simulink library "halout"  (R2021b)
settings: Solver=VariableStepAuto  StartTime=0.0  StopTime=10.0  RelTol=1e-3
undefined symbols (not defined in the file): C_TASK_5MS_S, FALSE, KHAL_CAN1FDAPS3E2E_flg, KHAL_CAN1FDAPS3TxReq_flg, KHAL_CAN1FDVCU2E2E_flg, KHAL_CAN1FDVCU2TxReq_flg, KHAL_CAN1FDVCU3E2E_flg, KHAL_CAN1FDVCU3TxReq_flg, KHAL_CAN1TxReq_flg, KHAL_CAN2TxReq_flg, KHAL_CAN3FDVCU1TxReq_flg, KHAL_CAN3FDVCU2E2E_flg, KHAL_CAN3FDVCU2TxReq_flg, KHAL_CAN3TxReq_flg, KHAL_CAN4FDVCU1E2E_flg, KHAL_CAN4FDVCU1TxReq_flg, KHAL_CAN4TxReq_flg, KHAL_CAN5TxReq_flg, ONE_INT, TRUE, ZERO_INT
libraries: FVT_lib x383, simulink x179
(part 10 of 20)

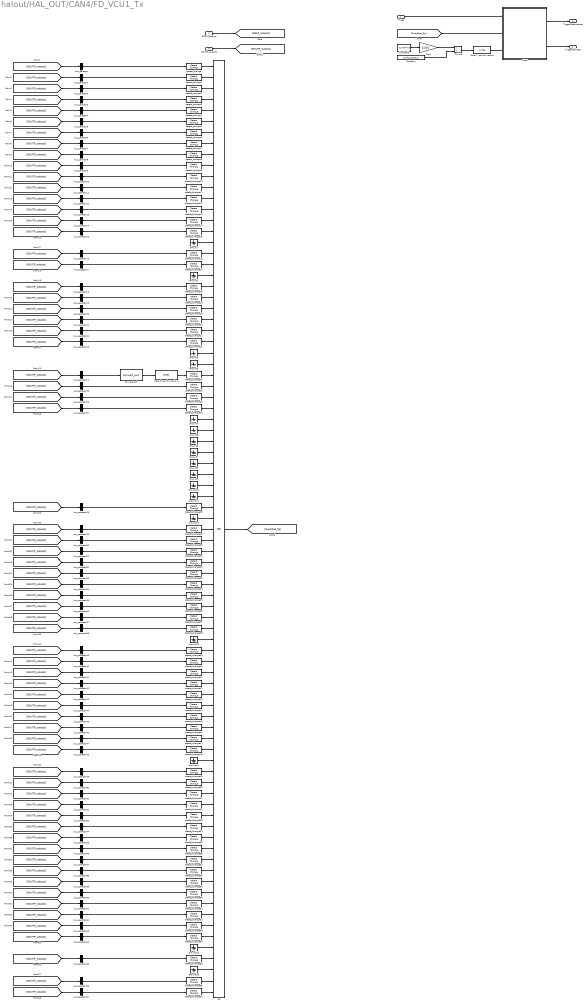
== system halout/HAL_OUT/CAN4/FD_VCU1_Tx ==
  TxReq : Inport
  BSCP_outputs : Inport  Port=2  OutDataTypeStr=Bus: BSCP_outputs
  BOUTP_outputs : Inport  Port=3  OutDataTypeStr=Bus: BOUTP_outputs
  Chart : Stateflow chart  TreatAsAtomicUnit=on
  Constant : Constant  Value=C_TASK_5MS_S
  Constant3 : Constant  Value=CycleTime
  Data Type Conversion : DataTypeConversion  OutDataTypeStr=uint16
  Data Type Conversion1 : DataTypeConversion  OutDataTypeStr=uint8
  Divide : Product  Inputs=*/
  Gain : Gain  Gain=0.001
  Ground{,1..16} (17 alike) : Ground
  OR : Logic  Operator=OR  Inputs=85  AllPortsSameDT=off  OutDataTypeStr=boolean
  bus_selector : BusSelector  OutputSignals=VOUTP_AllDoorSW_flg
  bus_selector1 : BusSelector  OutputSignals=VOUTP_AmbLightBreath1_flg
  bus_selector10 : BusSelector  OutputSignals=VOUTP_AntitheftSeatFlod_flg
  bus_selector11 : BusSelector  OutputSignals=VOUTP_AntitheftSta_enum
  bus_selector12 : BusSelector  OutputSignals=VOUTP_BCMBuzzerReq_flg
  bus_selector13 : BusSelector  OutputSignals=VOUTP_BCMDoorLockSta_flg
  bus_selector14 : BusSelector  OutputSignals=VOUTP_BrakeLamp_flg
  bus_selector15 : BusSelector  OutputSignals=VOUTP_CCCtrlSta_enum
  bus_selector16 : BusSelector  OutputSignals=VOUTP_CTDCtrl_enum
  bus_selector17 : BusSelector  OutputSignals=VOUTP_CTDLockSW_flg
  bus_selector18 : BusSelector  OutputSignals=VOUTP_CrashDetd_flg
  bus_selector19 : BusSelector  OutputSignals=VOUTP_CtrlDrPwrStbA2_flg
  bus_selector2 : BusSelector  OutputSignals=VOUTP_AmbLightBreath2_flg
  bus_selector20 : BusSelector  OutputSignals=VOUTP_CtrlFrBMSCCUCIR_flg
  bus_selector21 : BusSelector  OutputSignals=VOUTP_CtrlFrEDUINVERTER_flg
  bus_selector22 : BusSelector  OutputSignals=VOUTP_CtrlFrRC1_flg
  bus_selector23 : BusSelector  OutputSignals=VOUTP_CtrlFrPwrStbA1P_flg
  bus_selector24 : BusSelector  OutputSignals=VOUTP_Dimmer_pct
  bus_selector25 : BusSelector  OutputSignals=VOUTP_DimmerEN_flg
  bus_selector26 : BusSelector  OutputSignals=VOUTP_DoorLockIND_flg
  bus_selector27 : BusSelector  OutputSignals=VOUTP_DrDoorSW_flg
  bus_selector28 : BusSelector  OutputSignals=VOUTP_FrChargingDoorCtrl_enum
  bus_selector29 : BusSelector  OutputSignals=VOUTP_FrWiperH_flg
  bus_selector3 : BusSelector  OutputSignals=VOUTP_AmbLightBreath3_flg
  bus_selector30 : BusSelector  OutputSignals=VOUTP_FrWiperL_flg
  bus_selector31 : BusSelector  OutputSignals=VOUTP_HWResetSta_enum
  bus_selector32 : BusSelector  OutputSignals=VOUTP_HBeam_flg
  bus_selector33 : BusSelector  OutputSignals=VOUTP_HazardSW_flg
  bus_selector34 : BusSelector  OutputSignals=VOUTP_HoodSW_flg
  bus_selector35 : BusSelector  OutputSignals=VOUTP_HornCtrl_flg
  bus_selector36 : BusSelector  OutputSignals=VOUTP_LBSD_flg
  bus_selector37 : BusSelector  OutputSignals=VOUTP_LDRL_flg
  bus_selector38 : BusSelector  OutputSignals=VOUTP_LTurnLP_flg
  bus_selector39 : BusSelector  OutputSignals=VOUTP_LBeam_flg
  bus_selector4 : BusSelector  OutputSignals=VOUTP_AmbLightBrightness1_enum
  bus_selector40 : BusSelector  OutputSignals=VOUTP_LampPwr_flg
  bus_selector41 : BusSelector  OutputSignals=VOUTP_LockSetting_flg
  bus_selector42 : BusSelector  OutputSignals=VOUTP_MSACtrlSta_enum
  bus_selector43 : BusSelector  OutputSignals=VOUTP_MirrorCtrl_enum
  bus_selector44 : BusSelector  OutputSignals=VOUTP_MirrorDefog_flg
  bus_selector45 : BusSelector  OutputSignals=VOUTP_PosLamp_flg
  bus_selector46 : BusSelector  OutputSignals=VOUTP_PsDoorSW_flg
  bus_selector47 : BusSelector  OutputSignals=VOUTP_PowerSta_enum
  bus_selector48 : BusSelector  OutputSignals=VOUTP_RBSD_flg
  bus_selector49 : BusSelector  OutputSignals=VOUTP_RDRL_flg
  bus_selector5 : BusSelector  OutputSignals=VOUTP_AmbLightBrightness2_enum
  bus_selector50 : BusSelector  OutputSignals=VOUTP_RLDoorSW_flg
  bus_selector51 : BusSelector  OutputSignals=VOUTP_RRDoorSW_flg
  bus_selector52 : BusSelector  OutputSignals=VOUTP_RTurnLP_flg
  bus_selector53 : BusSelector  OutputSignals=VOUTP_ReBrakeLPReq_flg
  bus_selector54 : BusSelector  OutputSignals=VOUTP_ReverseLamp_flg
  bus_selector55 : BusSelector  OutputSignals=VOUTP_RoomLampH_flg
  bus_selector56 : BusSelector  OutputSignals=VOUTP_RoomLampL_flg
  bus_selector57 : BusSelector  OutputSignals=VOUTP_RrChargingDoorCtrl_enum
  bus_selector58 : BusSelector  OutputSignals=VOUTP_RrDefog_flg
  bus_selector59 : BusSelector  OutputSignals=VOUTP_RrFogLamp_flg
  bus_selector6 : BusSelector  OutputSignals=VOUTP_AmbLightBrightness3_enum
  bus_selector60 : BusSelector  OutputSignals=VOUTP_RrWiper_flg
  bus_selector61 : BusSelector  OutputSignals=VOUTP_ShiftGearPosn_enum
  bus_selector62 : BusSelector  OutputSignals=VOUTP_TailgateHDSW_flg
  bus_selector63 : BusSelector  OutputSignals=VOUTP_TailgateRemote_enum
  bus_selector64 : BusSelector  OutputSignals=VOUTP_TailgateSW_flg
  bus_selector65 : BusSelector  OutputSignals=VOUTP_TrunkRel_flg
  bus_selector66 : BusSelector  OutputSignals=VOUTP_WasherCtrl_enum
  bus_selector67 : BusSelector  OutputSignals=VOUTP_WiperFixMode_flg
  bus_selector7 : BusSelector  OutputSignals=VOUTP_AmbLightColor1_enum
  bus_selector8 : BusSelector  OutputSignals=VOUTP_AmbLightColor2_enum
  bus_selector9 : BusSelector  OutputSignals=VOUTP_AmbLightColor3_enum
  convert_out : FVT_lib/hal/convert_out  gain=1  offset=0
  detect_change{,1..67} (68 alike) : simulink/Logic and Bit Operations/Detect Change  vinit=0  OutDataTypeStr=boolean
  TriggerDataUpdate : Outport
  TriggerCallCDD : Outport  Port=2
  wires:
  Data Type Conversion/1 -> Chart/3(CycleCnt)
  TxReq/1 -> Chart/1(TxReq)
  [EventReq_flg] -> Chart/2(EventReq)
  Constant/1 -> Divide/2
  Divide/1 -> Data Type Conversion/1
  Gain/1 -> Divide/1
  Constant3/1 -> Gain/1
  BSCP_outputs/1 -> [BSCP_outputs]
  BOUTP_outputs/1 -> [BOUTP_outputs]
  OR/1 -> [EventReq_flg]
  detect_change/1 -> OR/1
  bus_selector/1 -> detect_change/1  "<VOUTP_AllDoorSW_flg>"
  [BOUTP_outputs] -> bus_selector/1
  detect_change1/1 -> OR/2
  bus_selector1/1 -> detect_change1/1  "<VOUTP_AmbLightBreath1_flg>"
  [BOUTP_outputs] -> bus_selector1/1
  detect_change2/1 -> OR/3
  bus_selector2/1 -> detect_change2/1  "<VOUTP_AmbLightBreath2_flg>"
  [BOUTP_outputs] -> bus_selector2/1
  detect_change3/1 -> OR/4
  bus_selector3/1 -> detect_change3/1  "<VOUTP_AmbLightBreath3_flg>"
  [BOUTP_outputs] -> bus_selector3/1
  detect_change4/1 -> OR/5
  bus_selector4/1 -> detect_change4/1  "<VOUTP_AmbLightBrightness1_enum>"
  [BOUTP_outputs] -> bus_selector4/1
  detect_change5/1 -> OR/6
  bus_selector5/1 -> detect_change5/1  "<VOUTP_AmbLightBrightness2_enum>"
  [BOUTP_outputs] -> bus_selector5/1
  detect_change6/1 -> OR/7
  bus_selector6/1 -> detect_change6/1  "<VOUTP_AmbLightBrightness3_enum>"
  [BOUTP_outputs] -> bus_selector6/1
  detect_change7/1 -> OR/8
  bus_selector7/1 -> detect_change7/1  "<VOUTP_AmbLightColor1_enum>"
  [BOUTP_outputs] -> bus_selector7/1
  detect_change8/1 -> OR/9
  bus_selector8/1 -> detect_change8/1  "<VOUTP_AmbLightColor2_enum>"
  [BOUTP_outputs] -> bus_selector8/1
  detect_change9/1 -> OR/10
  bus_selector9/1 -> detect_change9/1  "<VOUTP_AmbLightColor3_enum>"
  [BOUTP_outputs] -> bus_selector9/1
  detect_change10/1 -> OR/11
  bus_selector10/1 -> detect_change10/1  "<VOUTP_AntitheftSeatFlod_flg>"
  [BOUTP_outputs] -> bus_selector10/1
  detect_change11/1 -> OR/12
  bus_selector11/1 -> detect_change11/1  "<VOUTP_AntitheftSta_enum>"
  [BOUTP_outputs] -> bus_selector11/1
  detect_change12/1 -> OR/13
  bus_selector12/1 -> detect_change12/1  "<VOUTP_BCMBuzzerReq_flg>"
  [BOUTP_outputs] -> bus_selector12/1
  detect_change13/1 -> OR/14
  bus_selector13/1 -> detect_change13/1  "<VOUTP_BCMDoorLockSta_flg>"
  [BOUTP_outputs] -> bus_selector13/1
  detect_change14/1 -> OR/15
  bus_selector14/1 -> detect_change14/1  "<VOUTP_BrakeLamp_flg>"
  [BOUTP_outputs] -> bus_selector14/1
  detect_change15/1 -> OR/16
  bus_selector15/1 -> detect_change15/1  "<VOUTP_CCCtrlSta_enum>"
  [BOUTP_outputs] -> bus_selector15/1
  Ground/1 -> OR/17
  detect_change16/1 -> OR/18
  bus_selector16/1 -> detect_change16/1  "<VOUTP_CTDCtrl_enum>"
  [BOUTP_outputs] -> bus_selector16/1
  detect_change17/1 -> OR/19
  bus_selector17/1 -> detect_change17/1  "<VOUTP_CTDLockSW_flg>"
  [BOUTP_outputs] -> bus_selector17/1
  Ground1/1 -> OR/20
  detect_change18/1 -> OR/21
  bus_selector18/1 -> detect_change18/1  "<VOUTP_CrashDetd_flg>"
  [BOUTP_outputs] -> bus_selector18/1
  detect_change19/1 -> OR/22
  bus_selector19/1 -> detect_change19/1  "<VOUTP_CtrlDrPwrStbA2_flg>"
  [BOUTP_outputs] -> bus_selector19/1
  detect_change20/1 -> OR/23
  bus_selector20/1 -> detect_change20/1  "<VOUTP_CtrlFrBMSCCUCIR_flg>"
  [BOUTP_outputs] -> bus_selector20/1
  detect_change21/1 -> OR/24
  bus_selector21/1 -> detect_change21/1  "<VOUTP_CtrlFrEDUINVERTER_flg>"
  [BOUTP_outputs] -> bus_selector21/1
  detect_change22/1 -> OR/25
  bus_selector22/1 -> detect_change22/1  "<VOUTP_CtrlFrRC1_flg>"
  [BOUTP_outputs] -> bus_selector22/1
  detect_change23/1 -> OR/26
  bus_selector23/1 -> detect_change23/1  "<VOUTP_CtrlFrPwrStbA1P_flg>"
  [BOUTP_outputs] -> bus_selector23/1
  Ground2/1 -> OR/27
  Ground3/1 -> OR/28
  detect_change24/1 -> OR/29
  Data Type Conversion1/1 -> detect_change24/1
  convert_out/1 -> Data Type Conversion1/1
  bus_selector24/1 -> convert_out/1  "<VOUTP_Dimmer_pct>"
  [BOUTP_outputs] -> bus_selector24/1
  detect_change25/1 -> OR/30
  bus_selector25/1 -> detect_change25/1  "<VOUTP_DimmerEN_flg>"
  [BOUTP_outputs] -> bus_selector25/1
  detect_change26/1 -> OR/31
  bus_selector26/1 -> detect_change26/1  "<VOUTP_DoorLockIND_flg>"
  [BOUTP_outputs] -> bus_selector26/1
  detect_change27/1 -> OR/32
  bus_selector27/1 -> detect_change27/1  "<VOUTP_DrDoorSW_flg>"
  [BOUTP_outputs] -> bus_selector27/1
  Ground4/1 -> OR/33
  Ground5/1 -> OR/34
  Ground6/1 -> OR/35
  Ground7/1 -> OR/36
  Ground8/1 -> OR/37
  Ground9/1 -> OR/38
  Ground10/1 -> OR/39
  Ground11/1 -> OR/40
  detect_change28/1 -> OR/41
  bus_selector28/1 -> detect_change28/1  "<VOUTP_FrChargingDoorCtrl_enum>"
  [BOUTP_outputs] -> bus_selector28/1
  Ground12/1 -> OR/42
  detect_change29/1 -> OR/43
  bus_selector29/1 -> detect_change29/1  "<VOUTP_FrWiperH_flg>"
  [BOUTP_outputs] -> bus_selector29/1
  detect_change30/1 -> OR/44
  bus_selector30/1 -> detect_change30/1  "<VOUTP_FrWiperL_flg>"
  [BOUTP_outputs] -> bus_selector30/1
  detect_change31/1 -> OR/45
  bus_selector31/1 -> detect_change31/1  "<VOUTP_HWResetSta_enum>"
  [BOUTP_outputs] -> bus_selector31/1
  detect_change32/1 -> OR/46
  bus_selector32/1 -> detect_change32/1  "<VOUTP_HBeam_flg>"
  [BOUTP_outputs] -> bus_selector32/1
  detect_change33/1 -> OR/47
  bus_selector33/1 -> detect_change33/1  "<VOUTP_HazardSW_flg>"
  [BOUTP_outputs] -> bus_selector33/1
  detect_change34/1 -> OR/48
  bus_selector34/1 -> detect_change34/1  "<VOUTP_HoodSW_flg>"
  [BOUTP_outputs] -> bus_selector34/1
  detect_change35/1 -> OR/49
  bus_selector35/1 -> detect_change35/1  "<VOUTP_HornCtrl_flg>"
  [BOUTP_outputs] -> bus_selector35/1
  detect_change36/1 -> OR/50
  bus_selector36/1 -> detect_change36/1  "<VOUTP_LBSD_flg>"
  [BOUTP_outputs] -> bus_selector36/1
  detect_change37/1 -> OR/51
  bus_selector37/1 -> detect_change37/1  "<VOUTP_LDRL_flg>"
  [BOUTP_outputs] -> bus_selector37/1
  detect_change38/1 -> OR/52
  bus_selector38/1 -> detect_change38/1  "<VOUTP_LTurnLP_flg>"
  [BOUTP_outputs] -> bus_selector38/1
  Ground13/1 -> OR/53
  detect_change39/1 -> OR/54
  bus_selector39/1 -> detect_change39/1  "<VOUTP_LBeam_flg>"
  [BOUTP_outputs] -> bus_selector39/1
  detect_change40/1 -> OR/55
  bus_selector40/1 -> detect_change40/1  "<VOUTP_LampPwr_flg>"
  [BOUTP_outputs] -> bus_selector40/1
  detect_change41/1 -> OR/56
  bus_selector41/1 -> detect_change41/1  "<VOUTP_LockSetting_flg>"
  [BOUTP_outputs] -> bus_selector41/1
  detect_change42/1 -> OR/57
  bus_selector42/1 -> detect_change42/1  "<VOUTP_MSACtrlSta_enum>"
  [BOUTP_outputs] -> bus_selector42/1
  detect_change43/1 -> OR/58
  bus_selector43/1 -> detect_change43/1  "<VOUTP_MirrorCtrl_enum>"
  [BOUTP_outputs] -> bus_selector43/1
  detect_change44/1 -> OR/59
  bus_selector44/1 -> detect_change44/1  "<VOUTP_MirrorDefog_flg>"
  [BOUTP_outputs] -> bus_selector44/1
  detect_change45/1 -> OR/60
  bus_selector45/1 -> detect_change45/1  "<VOUTP_PosLamp_flg>"
  [BOUTP_outputs] -> bus_selector45/1
  detect_change46/1 -> OR/61
  bus_selector46/1 -> detect_change46/1  "<VOUTP_PsDoorSW_flg>"
  [BOUTP_outputs] -> bus_selector46/1
  detect_change47/1 -> OR/62
  bus_selector47/1 -> detect_change47/1  "<VOUTP_PowerSta_enum>"
  [BOUTP_outputs] -> bus_selector47/1
  detect_change48/1 -> OR/63
  bus_selector48/1 -> detect_change48/1  "<VOUTP_RBSD_flg>"
  [BOUTP_outputs] -> bus_selector48/1
  Ground14/1 -> OR/64
  detect_change49/1 -> OR/65
  bus_selector49/1 -> detect_change49/1  "<VOUTP_RDRL_flg>"
  [BOUTP_outputs] -> bus_selector49/1
  detect_change50/1 -> OR/66
  bus_selector50/1 -> detect_change50/1  "<VOUTP_RLDoorSW_flg>"
  [BOUTP_outputs] -> bus_selector50/1
  detect_change51/1 -> OR/67
  bus_selector51/1 -> detect_change51/1  "<VOUTP_RRDoorSW_flg>"
  [BOUTP_outputs] -> bus_selector51/1
  detect_change52/1 -> OR/68
  bus_selector52/1 -> detect_change52/1  "<VOUTP_RTurnLP_flg>"
  [BOUTP_outputs] -> bus_selector52/1
  detect_change53/1 -> OR/69
  bus_selector53/1 -> detect_change53/1  "<VOUTP_ReBrakeLPReq_flg>"
  [BOUTP_outputs] -> bus_selector53/1
  detect_change54/1 -> OR/70
  bus_selector54/1 -> detect_change54/1  "<VOUTP_ReverseLamp_flg>"
  [BOUTP_outputs] -> bus_selector54/1
  detect_change55/1 -> OR/71
  bus_selector55/1 -> detect_change55/1  "<VOUTP_RoomLampH_flg>"
  [BOUTP_outputs] -> bus_selector55/1
  detect_change56/1 -> OR/72
  bus_selector56/1 -> detect_change56/1  "<VOUTP_RoomLampL_flg>"
  [BOUTP_outputs] -> bus_selector56/1
  detect_change57/1 -> OR/73
  bus_selector57/1 -> detect_change57/1  "<VOUTP_RrChargingDoorCtrl_enum>"
  [BOUTP_outputs] -> bus_selector57/1
  detect_change58/1 -> OR/74
  bus_selector58/1 -> detect_change58/1  "<VOUTP_RrDefog_flg>"
  [BOUTP_outputs] -> bus_selector58/1
  detect_change59/1 -> OR/75
  bus_selector59/1 -> detect_change59/1  "<VOUTP_RrFogLamp_flg>"
  [BOUTP_outputs] -> bus_selector59/1
  detect_change60/1 -> OR/76
  bus_selector60/1 -> detect_change60/1  "<VOUTP_RrWiper_flg>"
  [BOUTP_outputs] -> bus_selector60/1
  detect_change61/1 -> OR/77
  bus_selector61/1 -> detect_change61/1  "<VOUTP_ShiftGearPosn_enum>"
  [BOUTP_outputs] -> bus_selector61/1
  detect_change62/1 -> OR/78
  bus_selector62/1 -> detect_change62/1  "<VOUTP_TailgateHDSW_flg>"
  [BOUTP_outputs] -> bus_selector62/1
  detect_change63/1 -> OR/79
  bus_selector63/1 -> detect_change63/1  "<VOUTP_TailgateRemote_enum>"
  [BOUTP_outputs] -> bus_selector63/1
  detect_change64/1 -> OR/80
  bus_selector64/1 -> detect_change64/1  "<VOUTP_TailgateSW_flg>"
  [BOUTP_outputs] -> bus_selector64/1
  Ground15/1 -> OR/81
  detect_change65/1 -> OR/82
  bus_selector65/1 -> detect_change65/1  "<VOUTP_TrunkRel_flg>"
  [BOUTP_outputs] -> bus_selector65/1
  Ground16/1 -> OR/83
  detect_change66/1 -> OR/84
  bus_selector66/1 -> detect_change66/1  "<VOUTP_WasherCtrl_enum>"
  [BOUTP_outputs] -> bus_selector66/1
  detect_change67/1 -> OR/85
  bus_selector67/1 -> detect_change67/1  "<VOUTP_WiperFixMode_flg>"
  [BOUTP_outputs] -> bus_selector67/1
  Chart/1(TriggerDataUpdate()) -> TriggerDataUpdate/1
  Chart/2(TriggerCallCDD()) -> TriggerCallCDD/1

== system halout/HAL_OUT/CAN4/Function-Call Subsystem ==
  function : TriggerPort  TriggerType=function-call  VariantControl=(inherit)
  Add : Sum
  Constant : Constant  Value=ONE_INT
  Constant1 : Constant  Value=ZERO_INT
  Constant2 : Constant  Value=uint8(10)
  GreaterThan : RelationalOperator  Operator=>  OutDataTypeStr=boolean  RndMeth=Simplest
  Switch : Switch  Criteria=u2 ~= 0
  Unit Delay : UnitDelay  SampleTime=-1  HasFrameUpgradeWarning=on
  TriggerCAN4VCU1_CNT : Outport
  wires:
  Add/1 -> Switch/3, GreaterThan/1
  Unit Delay/1 -> Add/1
  Constant/1 -> Add/2
  Switch/1 -> TriggerCAN4VCU1_CNT/1, Unit Delay/1
  Constant2/1 -> GreaterThan/2
  GreaterThan/1 -> Switch/2
  Constant1/1 -> Switch/1

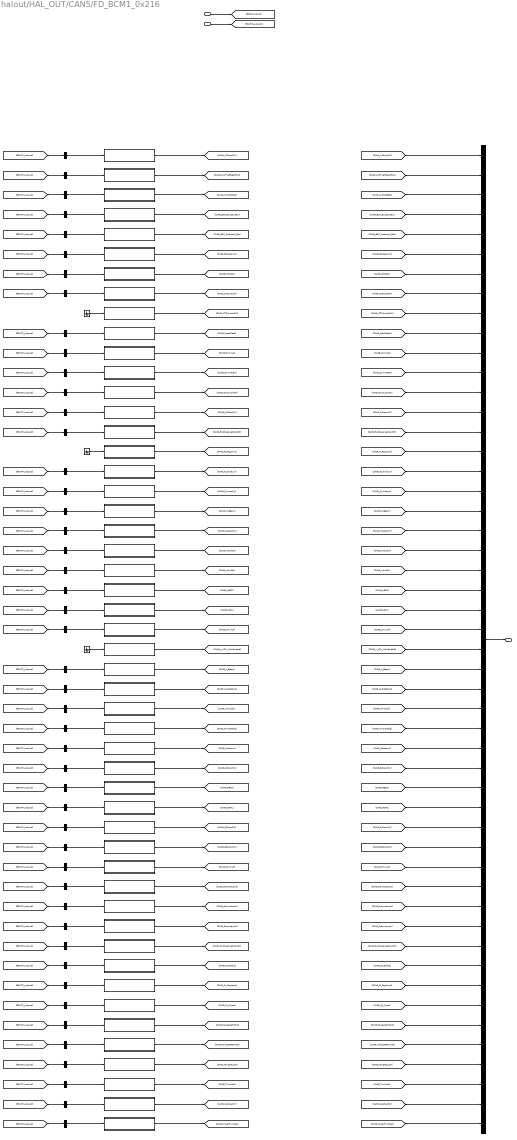
== system halout/HAL_OUT/CAN5/FD_BCM1_0x216 ==
  BSCP_outputs : Inport  OutDataTypeStr=Bus: BSCP_outputs
  BOUTP_outputs : Inport  Port=2  OutDataTypeStr=Bus: BOUTP_outputs
  AllDoorSW : Subsystem
  AntiTheftSeatFold : Subsystem
  AntitheftSta : Subsystem
  BCMBuzzerReq : Subsystem
  BCMDoorLockSta : Subsystem
  BrakeLamp : Subsystem
  CTDCtrl : Subsystem
  CTDLockSW : Subsystem
  CTDUnlockSW : Subsystem
  CrashDetd : Subsystem
  Dimmer : Subsystem
  DimmerEN : Subsystem
  DoorLockIND : Subsystem
  DrDoorSW : Subsystem
  FrChargingDoorCtrl : Subsystem
  FrFogLamp : Subsystem
  FrWiperH : Subsystem
  FrWiperL : Subsystem
  Ground : Ground
  Ground1 : Ground
  Ground2 : Ground
  HBeam : Subsystem
  HazardSW : Subsystem
  HoodSW : Subsystem
  HornCtrl : Subsystem
  LAPMWdwEnable : Subsystem
  LBSD : Subsystem
  LBeam : Subsystem
  LDRL : Subsystem
  LTurnLP : Subsystem
  LockSetting : Subsystem
  MirrorCtrl : Subsystem
  MirrorDefog : Subsystem
  PosLamp : Subsystem
  PsDoorSW : Subsystem
  RBSD : Subsystem
  RDRL : Subsystem
  RLDoorSW : Subsystem
  RRDoorSW : Subsystem
  RTurnLP : Subsystem
  ReverseLamp : Subsystem
  RoomLampH : Subsystem
  RoomLampL : Subsystem
  RrChargingDoorCtrl : Subsystem
  RrDefog : Subsystem
  RrFogLamp : Subsystem
  RrWiper : Subsystem
  TailgateHDSW : Subsystem
  TailgateRemote : Subsystem
  TailgateSW : Subsystem
  TrunkRel : Subsystem
  WasherCtrl : Subsystem
  WiperFixMode : Subsystem
  bus_creator : BusCreator  Inputs=50  OutDataTypeStr=Bus: DT_CAN5_SG_FD_BCM1  NonVirtualBus=on
  bus_selector : BusSelector  OutputSignals=VOUTP_AllDoorSW_flg
  bus_selector1 : BusSelector  OutputSignals=VOUTP_AntitheftSeatFlod_flg
  bus_selector10 : BusSelector  OutputSignals=VOUTP_DimmerEN_flg
  bus_selector11 : BusSelector  OutputSignals=VOUTP_DoorLockIND_flg
  bus_selector12 : BusSelector  OutputSignals=VOUTP_DrDoorSW_flg
  bus_selector13 : BusSelector  OutputSignals=VOUTP_FrChargingDoorCtrl_enum
  bus_selector14 : BusSelector  OutputSignals=VOUTP_FrWiperH_flg
  bus_selector15 : BusSelector  OutputSignals=VOUTP_FrWiperL_flg
  bus_selector16 : BusSelector  OutputSignals=VOUTP_HBeam_flg
  bus_selector17 : BusSelector  OutputSignals=VOUTP_HazardSW_flg
  bus_selector18 : BusSelector  OutputSignals=VOUTP_HoodSW_flg
  bus_selector19 : BusSelector  OutputSignals=VOUTP_HornCtrl_flg
  bus_selector2 : BusSelector  OutputSignals=VOUTP_AntitheftSta_enum
  bus_selector20 : BusSelector  OutputSignals=VOUTP_LBSD_flg
  bus_selector21 : BusSelector  OutputSignals=VOUTP_LDRL_flg
  bus_selector22 : BusSelector  OutputSignals=VOUTP_LTurnLP_flg
  bus_selector23 : BusSelector  OutputSignals=VOUTP_LBeam_flg
  bus_selector24 : BusSelector  OutputSignals=VOUTP_LockSetting_flg
  bus_selector25 : BusSelector  OutputSignals=VOUTP_MirrorCtrl_enum
  bus_selector26 : BusSelector  OutputSignals=VOUTP_MirrorDefog_flg
  bus_selector27 : BusSelector  OutputSignals=VOUTP_PosLamp_flg
  bus_selector28 : BusSelector  OutputSignals=VOUTP_PsDoorSW_flg
  bus_selector29 : BusSelector  OutputSignals=VOUTP_RBSD_flg
  bus_selector3 : BusSelector  OutputSignals=VOUTP_BCMBuzzerReq_flg
  bus_selector30 : BusSelector  OutputSignals=VOUTP_RDRL_flg
  bus_selector31 : BusSelector  OutputSignals=VOUTP_RLDoorSW_flg
  bus_selector32 : BusSelector  OutputSignals=VOUTP_RRDoorSW_flg
  bus_selector33 : BusSelector  OutputSignals=VOUTP_RTurnLP_flg
  bus_selector34 : BusSelector  OutputSignals=VOUTP_ReverseLamp_flg
  bus_selector35 : BusSelector  OutputSignals=VOUTP_RoomLampH_flg
  bus_selector36 : BusSelector  OutputSignals=VOUTP_RoomLampL_flg
  bus_selector37 : BusSelector  OutputSignals=VOUTP_RrChargingDoorCtrl_enum
  bus_selector38 : BusSelector  OutputSignals=VOUTP_RrDefog_flg
  bus_selector39 : BusSelector  OutputSignals=VOUTP_RrFogLamp_flg
  bus_selector4 : BusSelector  OutputSignals=VOUTP_BCMDoorLockSta_flg
  bus_selector40 : BusSelector  OutputSignals=VOUTP_RrWiper_flg
  bus_selector41 : BusSelector  OutputSignals=VOUTP_TailgateHDSW_flg
  bus_selector42 : BusSelector  OutputSignals=VOUTP_TailgateRemote_enum
  bus_selector43 : BusSelector  OutputSignals=VOUTP_TailgateSW_flg
  bus_selector44 : BusSelector  OutputSignals=VOUTP_TrunkRel_flg
  bus_selector45 : BusSelector  OutputSignals=VOUTP_WasherCtrl_enum
  bus_selector46 : BusSelector  OutputSignals=VOUTP_WiperFixMode_flg
  bus_selector5 : BusSelector  OutputSignals=VOUTP_BrakeLamp_flg
  bus_selector6 : BusSelector  OutputSignals=VOUTP_CTDCtrl_enum
  bus_selector7 : BusSelector  OutputSignals=VOUTP_CTDLockSW_flg
  bus_selector8 : BusSelector  OutputSignals=VOUTP_CrashDetd_flg
  bus_selector9 : BusSelector  OutputSignals=VOUTP_Dimmer_pct
  FD_BCM1 : Outport
  wires:
  BSCP_outputs/1 -> [BSCP_outputs]
  BOUTP_outputs/1 -> [BOUTP_outputs]
  [CAN5_AllDoorSW] -> bus_creator/1  "CAN5_AllDoorSW"
  [CAN5_AntiTheftSeatFold] -> bus_creator/2  "CAN5_AntiTheftSeatFold"
  [CAN5_AntitheftSta] -> bus_creator/3  "CAN5_AntitheftSta"
  [CAN5_BCM_Buzzer_Req] -> bus_creator/4  "CAN5_BCM_Buzzer_Req"
  [CAN5_BCM_DoorLock_Sta] -> bus_creator/5  "CAN5_BCM_DoorLock_Sta"
  [CAN5_BrakeLamp] -> bus_creator/6  "CAN5_BrakeLamp"
  [CAN5_CTDCtrl] -> bus_creator/7  "CAN5_CTDCtrl"
  [CAN5_CTDLockSW] -> bus_creator/8  "CAN5_CTDLockSW"
  [CAN5_CTDUnlockSW] -> bus_creator/9  "CAN5_CTDUnlockSW"
  [CAN5_CrashDetd] -> bus_creator/10  "CAN5_CrashDetd"
  [CAN5_Dimmer] -> bus_creator/11  "CAN5_Dimmer"
  [CAN5_DimmerEN] -> bus_creator/12  "CAN5_DimmerEN"
  [CAN5_DoorLockIND] -> bus_creator/13  "CAN5_DoorLockIND"
  [CAN5_DrDoorSW] -> bus_creator/14  "CAN5_DrDoorSW"
  [CAN5_Fr_ChargingDoorCtrl] -> bus_creator/15  "CAN5_Fr_ChargingDoorCtrl"
  [CAN5_Fr_FogLamp] -> bus_creator/16  "CAN5_Fr_FogLamp"
  [CAN5_Fr_Wiper_H] -> bus_creator/17  "CAN5_Fr_Wiper_H"
  [CAN5_Fr_Wiper_L] -> bus_creator/18  "CAN5_Fr_Wiper_L"
  [CAN5_H_Beam] -> bus_creator/19  "CAN5_H_Beam"
  [CAN5_HazardSW] -> bus_creator/20  "CAN5_HazardSW"
  [CAN5_HoodSW] -> bus_creator/21  "CAN5_HoodSW"
  [CAN5_HornCtrl] -> bus_creator/22  "CAN5_HornCtrl"
  [CAN5_LBSD] -> bus_creator/23  "CAN5_LBSD"
  [CAN5_LDRL] -> bus_creator/24  "CAN5_LDRL"
  [CAN5_LTurnLP] -> bus_creator/25  "CAN5_LTurnLP"
  [CAN5_L_APM_WdwEnable] -> bus_creator/26  "CAN5_L_APM_WdwEnable"
  [CAN5_L_Beam] -> bus_creator/27  "CAN5_L_Beam"
  [CAN5_LockSetting] -> bus_creator/28  "CAN5_LockSetting"
  [CAN5_MirrorCtrl] -> bus_creator/29  "CAN5_MirrorCtrl"
  [CAN5_MirrorDefog] -> bus_creator/30  "CAN5_MirrorDefog"
  [CAN5_PosLamp] -> bus_creator/31  "CAN5_PosLamp"
  [CAN5_PsDoorSW] -> bus_creator/32  "CAN5_PsDoorSW"
  [CAN5_RBSD] -> bus_creator/33  "CAN5_RBSD"
  [CAN5_RDRL] -> bus_creator/34  "CAN5_RDRL"
  [CAN5_RLDoorSW] -> bus_creator/35  "CAN5_RLDoorSW"
  [CAN5_RRDoorSW] -> bus_creator/36  "CAN5_RRDoorSW"
  [CAN5_RTurnLP] -> bus_creator/37  "CAN5_RTurnLP"
  [CAN5_ReverseLamp] -> bus_creator/38  "CAN5_ReverseLamp"
  [CAN5_RoomLampH] -> bus_creator/39  "CAN5_RoomLampH"
  [CAN5_RoomLampL] -> bus_creator/40  "CAN5_RoomLampL"
  [CAN5_Rr_ChargingDoorCtrl] -> bus_creator/41  "CAN5_Rr_ChargingDoorCtrl"
  [CAN5_Rr_Defog] -> bus_creator/42  "CAN5_Rr_Defog"
  [CAN5_Rr_FogLamp] -> bus_creator/43  "CAN5_Rr_FogLamp"
  [CAN5_Rr_Wiper] -> bus_creator/44  "CAN5_Rr_Wiper"
  [CAN5_TailgateHDSW] -> bus_creator/45  "CAN5_TailgateHDSW"
  [CAN5_TailgateRemote] -> bus_creator/46  "CAN5_TailgateRemote"
  [CAN5_Tailgate_SW] -> bus_creator/47  "CAN5_Tailgate_SW"
  [CAN5_TrunkRel] -> bus_creator/48  "CAN5_TrunkRel"
  [CAN5_WasherCtrl] -> bus_creator/49  "CAN5_WasherCtrl"
  [CAN5_WiperFixMode] -> bus_creator/50  "CAN5_WiperFixMode"
  bus_creator/1 -> FD_BCM1/1
  AllDoorSW/1(CAN5_AllDoorSW) -> [CAN5_AllDoorSW]
  AntiTheftSeatFold/1(CAN5_AntiTheftSeatFold) -> [CAN5_AntiTheftSeatFold]
  AntitheftSta/1(CAN5_AntitheftSta) -> [CAN5_AntitheftSta]
  BCMBuzzerReq/1(CAN5_BCM_Buzzer_Req) -> [CAN5_BCM_Buzzer_Req]
  BCMDoorLockSta/1(CAN5_BCM_DoorLock_Sta) -> [CAN5_BCM_DoorLock_Sta]
  BrakeLamp/1(CAN5_BrakeLamp) -> [CAN5_BrakeLamp]
  CTDCtrl/1(CAN5_CTDCtrl) -> [CAN5_CTDCtrl]
  CTDLockSW/1(CAN5_CTDLockSW) -> [CAN5_CTDLockSW]
  CTDUnlockSW/1(CAN5_CTDUnlockSW) -> [CAN5_CTDUnlockSW]
  CrashDetd/1(CAN5_CrashDetd) -> [CAN5_CrashDetd]
  Dimmer/1(CAN5_Dimmer) -> [CAN5_Dimmer]
  DimmerEN/1(CAN5_DimmerEN) -> [CAN5_DimmerEN]
  DoorLockIND/1(CAN5_DoorLockIND) -> [CAN5_DoorLockIND]
  DrDoorSW/1(CAN5_DrDoorSW) -> [CAN5_DrDoorSW]
  FrChargingDoorCtrl/1(CAN5_Fr_ChargingDoorCtrl) -> [CAN5_Fr_ChargingDoorCtrl]
  FrFogLamp/1(CAN5_Fr_FogLamp) -> [CAN5_Fr_FogLamp]
  FrWiperH/1(CAN5_Fr_Wiper_H) -> [CAN5_Fr_Wiper_H]
  FrWiperL/1(CAN5_Fr_Wiper_L) -> [CAN5_Fr_Wiper_L]
  HBeam/1(CAN5_H_Beam) -> [CAN5_H_Beam]
  HazardSW/1(CAN5_HazardSW) -> [CAN5_HazardSW]
  HoodSW/1(CAN5_HoodSW) -> [CAN5_HoodSW]
  HornCtrl/1(CAN5_HornCtrl) -> [CAN5_HornCtrl]
  LBSD/1(CAN5_LBSD) -> [CAN5_LBSD]
  LDRL/1(CAN5_LDRL) -> [CAN5_LDRL]
  LTurnLP/1(CAN5_LTurnLP) -> [CAN5_LTurnLP]
  LAPMWdwEnable/1(CAN5_L_APM_WdwEnable) -> [CAN5_L_APM_WdwEnable]
  LBeam/1(CAN5_L_Beam) -> [CAN5_L_Beam]
  LockSetting/1(CAN5_LockSetting) -> [CAN5_LockSetting]
  MirrorCtrl/1(CAN5_MirrorCtrl) -> [CAN5_MirrorCtrl]
  MirrorDefog/1(CAN5_MirrorDefog) -> [CAN5_MirrorDefog]
  PosLamp/1(CAN5_PosLamp) -> [CAN5_PosLamp]
  PsDoorSW/1(CAN5_PsDoorSW) -> [CAN5_PsDoorSW]
  RBSD/1(CAN5_RBSD) -> [CAN5_RBSD]
  RDRL/1(CAN5_RDRL) -> [CAN5_RDRL]
  RLDoorSW/1(CAN5_RLDoorSW) -> [CAN5_RLDoorSW]
  RRDoorSW/1(CAN5_RRDoorSW) -> [CAN5_RRDoorSW]
  RTurnLP/1(CAN5_RTurnLP) -> [CAN5_RTurnLP]
  ReverseLamp/1(CAN5_ReverseLamp) -> [CAN5_ReverseLamp]
  RoomLampH/1(CAN5_RoomLampH) -> [CAN5_RoomLampH]
  RoomLampL/1(CAN5_RoomLampL) -> [CAN5_RoomLampL]
  RrChargingDoorCtrl/1(CAN5_Rr_ChargingDoorCtrl) -> [CAN5_Rr_ChargingDoorCtrl]
  RrDefog/1(CAN5_Rr_Defog) -> [CAN5_Rr_Defog]
  RrFogLamp/1(CAN5_Rr_FogLamp) -> [CAN5_Rr_FogLamp]
  RrWiper/1(CAN5_Rr_Wiper) -> [CAN5_Rr_Wiper]
  TailgateHDSW/1(CAN5_TailgateHDSW) -> [CAN5_TailgateHDSW]
  TailgateRemote/1(CAN5_TailgateRemote) -> [CAN5_TailgateRemote]
  TailgateSW/1(CAN5_Tailgate_SW) -> [CAN5_Tailgate_SW]
  TrunkRel/1(CAN5_TrunkRel) -> [CAN5_TrunkRel]
  WasherCtrl/1(CAN5_WasherCtrl) -> [CAN5_WasherCtrl]
  WiperFixMode/1(CAN5_WiperFixMode) -> [CAN5_WiperFixMode]
  bus_selector/1 -> AllDoorSW/1(AllDoorSW)  "<VOUTP_AllDoorSW_flg>"
  [BOUTP_outputs] -> bus_selector/1
  bus_selector1/1 -> AntiTheftSeatFold/1(AntiTheftSeatFold)  "<VOUTP_AntitheftSeatFlod_flg>"
  [BOUTP_outputs] -> bus_selector1/1
  bus_selector2/1 -> AntitheftSta/1(AntitheftSta)  "<VOUTP_AntitheftSta_enum>"
  [BOUTP_outputs] -> bus_selector2/1
  bus_selector3/1 -> BCMBuzzerReq/1(BCMBuzzerReq)  "<VOUTP_BCMBuzzerReq_flg>"
  [BOUTP_outputs] -> bus_selector3/1
  bus_selector4/1 -> BCMDoorLockSta/1(BCMDoorLockSta)  "<VOUTP_BCMDoorLockSta_flg>"
  [BOUTP_outputs] -> bus_selector4/1
  bus_selector5/1 -> BrakeLamp/1(BrakeLamp)  "<VOUTP_BrakeLamp_flg>"
  [BOUTP_outputs] -> bus_selector5/1
  bus_selector6/1 -> CTDCtrl/1(CTDCtrl)  "<VOUTP_CTDCtrl_enum>"
  [BOUTP_outputs] -> bus_selector6/1
  bus_selector7/1 -> CTDLockSW/1(CTDLockSW)  "<VOUTP_CTDLockSW_flg>"
  [BOUTP_outputs] -> bus_selector7/1
  Ground/1 -> CTDUnlockSW/1(CTDUnlockSW)
  bus_selector8/1 -> CrashDetd/1(CrashDetd)  "<VOUTP_CrashDetd_flg>"
  [BOUTP_outputs] -> bus_selector8/1
  bus_selector9/1 -> Dimmer/1(Dimmer)  "<VOUTP_Dimmer_pct>"
  [BOUTP_outputs] -> bus_selector9/1
  bus_selector10/1 -> DimmerEN/1(DimmerEN)  "<VOUTP_DimmerEN_flg>"
  [BOUTP_outputs] -> bus_selector10/1
  bus_selector11/1 -> DoorLockIND/1(DoorLockIND)  "<VOUTP_DoorLockIND_flg>"
  [BOUTP_outputs] -> bus_selector11/1
  bus_selector12/1 -> DrDoorSW/1(DrDoorSW)  "<VOUTP_DrDoorSW_flg>"
  [BOUTP_outputs] -> bus_selector12/1
  bus_selector13/1 -> FrChargingDoorCtrl/1(FrChargingDoorCtrl)  "<VOUTP_FrChargingDoorCtrl_enum>"
  [BOUTP_outputs] -> bus_selector13/1
  Ground1/1 -> FrFogLamp/1(FrFogLamp)
  bus_selector14/1 -> FrWiperH/1(FrWiperH)  "<VOUTP_FrWiperH_flg>"
  [BOUTP_outputs] -> bus_selector14/1
  bus_selector15/1 -> FrWiperL/1(FrWiperL)  "<VOUTP_FrWiperL_flg>"
  [BOUTP_outputs] -> bus_selector15/1
  bus_selector16/1 -> HBeam/1(HBeam)  "<VOUTP_HBeam_flg>"
  [BOUTP_outputs] -> bus_selector16/1
  bus_selector17/1 -> HazardSW/1(HazardSW)  "<VOUTP_HazardSW_flg>"
  [BOUTP_outputs] -> bus_selector17/1
  bus_selector18/1 -> HoodSW/1(HoodSW)  "<VOUTP_HoodSW_flg>"
  [BOUTP_outputs] -> bus_selector18/1
  bus_selector19/1 -> HornCtrl/1(HornCtrl)  "<VOUTP_HornCtrl_flg>"
  [BOUTP_outputs] -> bus_selector19/1
  bus_selector20/1 -> LBSD/1(LBSD)  "<VOUTP_LBSD_flg>"
  [BOUTP_outputs] -> bus_selector20/1
  bus_selector21/1 -> LDRL/1(LDRL)  "<VOUTP_LDRL_flg>"
  [BOUTP_outputs] -> bus_selector21/1
  bus_selector22/1 -> LTurnLP/1(LTurnLP)  "<VOUTP_LTurnLP_flg>"
  [BOUTP_outputs] -> bus_selector22/1
  Ground2/1 -> LAPMWdwEnable/1(LAPMWdwEnable)
  bus_selector23/1 -> LBeam/1(LBeam)  "<VOUTP_LBeam_flg>"
  [BOUTP_outputs] -> bus_selector23/1
  bus_selector24/1 -> LockSetting/1(LockSetting)  "<VOUTP_LockSetting_flg>"
  [BOUTP_outputs] -> bus_selector24/1
  bus_selector25/1 -> MirrorCtrl/1(MirrorCtrl)  "<VOUTP_MirrorCtrl_enum>"
  [BOUTP_outputs] -> bus_selector25/1
  bus_selector26/1 -> MirrorDefog/1(MirrorDefog)  "<VOUTP_MirrorDefog_flg>"
  [BOUTP_outputs] -> bus_selector26/1
  bus_selector27/1 -> PosLamp/1(PosLamp)  "<VOUTP_PosLamp_flg>"
  [BOUTP_outputs] -> bus_selector27/1
  bus_selector28/1 -> PsDoorSW/1(PsDoorSW)  "<VOUTP_PsDoorSW_flg>"
  [BOUTP_outputs] -> bus_selector28/1
  bus_selector29/1 -> RBSD/1(RBSD)  "<VOUTP_RBSD_flg>"
  [BOUTP_outputs] -> bus_selector29/1
  bus_selector30/1 -> RDRL/1(RDRL)  "<VOUTP_RDRL_flg>"
  [BOUTP_outputs] -> bus_selector30/1
  bus_selector31/1 -> RLDoorSW/1(RLDoorSW)  "<VOUTP_RLDoorSW_flg>"
  [BOUTP_outputs] -> bus_selector31/1
  bus_selector32/1 -> RRDoorSW/1(RRDoorSW)  "<VOUTP_RRDoorSW_flg>"
  [BOUTP_outputs] -> bus_selector32/1
  bus_selector33/1 -> RTurnLP/1(RTurnLP)  "<VOUTP_RTurnLP_flg>"
  [BOUTP_outputs] -> bus_selector33/1
  bus_selector34/1 -> ReverseLamp/1(ReverseLamp)  "<VOUTP_ReverseLamp_flg>"
  [BOUTP_outputs] -> bus_selector34/1
  bus_selector35/1 -> RoomLampH/1(RoomLampH)  "<VOUTP_RoomLampH_flg>"
  [BOUTP_outputs] -> bus_selector35/1
  bus_selector36/1 -> RoomLampL/1(RoomLampL)  "<VOUTP_RoomLampL_flg>"
  [BOUTP_outputs] -> bus_selector36/1
  bus_selector37/1 -> RrChargingDoorCtrl/1(RrChargingDoorCtrl)  "<VOUTP_RrChargingDoorCtrl_enum>"
  [BOUTP_outputs] -> bus_selector37/1
  bus_selector38/1 -> RrDefog/1(RrDefog)  "<VOUTP_RrDefog_flg>"
  [BOUTP_outputs] -> bus_selector38/1
  bus_selector39/1 -> RrFogLamp/1(RrFogLamp)  "<VOUTP_RrFogLamp_flg>"
  [BOUTP_outputs] -> bus_selector39/1
  bus_selector40/1 -> RrWiper/1(RrWiper)  "<VOUTP_RrWiper_flg>"
  [BOUTP_outputs] -> bus_selector40/1
  bus_selector41/1 -> TailgateHDSW/1(TailgateHDSW)  "<VOUTP_TailgateHDSW_flg>"
  [BOUTP_outputs] -> bus_selector41/1
  bus_selector42/1 -> TailgateRemote/1(TailgateRemote)  "<VOUTP_TailgateRemote_enum>"
  [BOUTP_outputs] -> bus_selector42/1
  bus_selector43/1 -> TailgateSW/1(TailgateSW)  "<VOUTP_TailgateSW_flg>"
  [BOUTP_outputs] -> bus_selector43/1
  bus_selector44/1 -> TrunkRel/1(TrunkRel)  "<VOUTP_TrunkRel_flg>"
  [BOUTP_outputs] -> bus_selector44/1
  bus_selector45/1 -> WasherCtrl/1(WasherCtrl)  "<VOUTP_WasherCtrl_enum>"
  [BOUTP_outputs] -> bus_selector45/1
  bus_selector46/1 -> WiperFixMode/1(WiperFixMode)  "<VOUTP_WiperFixMode_flg>"
  [BOUTP_outputs] -> bus_selector46/1

== system halout/HAL_OUT/CAN5/FD_CONN1_0x43C ==
  BSCP_outputs : Inport  OutDataTypeStr=Bus: BSCP_outputs
  BOUTP_outputs : Inport  Port=2  OutDataTypeStr=Bus: BOUTP_outputs
  CCUAutoLampSts : Subsystem
  FDDKCVehDataErr : Subsystem
  FDDKCVehDataSta : Subsystem
  FDTBOXDTCDataErr : Subsystem
  FDTBOXDTCDataSta : Subsystem
  FDTBOXVehDataErr : Subsystem
  FDTBOXVehDataSta : Subsystem
  Ground{,1..5} (6 alike) : Ground
  SWCmodeSta : Subsystem
  bus_creator : BusCreator  Inputs=8  OutDataTypeStr=Bus: DT_CAN5_SG_FD_CONN1  NonVirtualBus=on
  bus_selector : BusSelector  OutputSignals=VOUTP_CCUAutoLampSts_flg
  bus_selector1 : BusSelector  OutputSignals=VSCP_CAN5FDCONN1SWCmodeSta_flg
  FD_CONN1 : Outport
  wires:
  BSCP_outputs/1 -> [BSCP_outputs]
  BOUTP_outputs/1 -> [BOUTP_outputs]
  [CAN5_CCU_AutoLampSts] -> bus_creator/1  "CAN5_CCU_AutoLampSts"
  [CAN5_FD_DKC_VehData_Err] -> bus_creator/2  "CAN5_FD_DKC_VehData_Err"
  [CAN5_FD_DKC_VehData_Sta] -> bus_creator/3  "CAN5_FD_DKC_VehData_Sta"
  [CAN5_FD_TBOX_DTCData_Err] -> bus_creator/4  "CAN5_FD_TBOX_DTCData_Err"
  [CAN5_FD_TBOX_DTCData_Sta] -> bus_creator/5  "CAN5_FD_TBOX_DTCData_Sta"
  [CAN5_FD_TBOX_VehData_Err] -> bus_creator/6  "CAN5_FD_TBOX_VehData_Err"
  [CAN5_FD_TBOX_VehData_Sta] -> bus_creator/7  "CAN5_FD_TBOX_VehData_Sta"
  [CAN5_SWC_mode_Sta] -> bus_creator/8  "CAN5_SWC_mode_Sta"
  bus_creator/1 -> FD_CONN1/1
  CCUAutoLampSts/1(CAN5_CCU_AutoLampSts) -> [CAN5_CCU_AutoLampSts]
  FDDKCVehDataErr/1(CAN5_FD_DKC_VehData_Err) -> [CAN5_FD_DKC_VehData_Err]
  FDDKCVehDataSta/1(CAN5_FD_DKC_VehData_Sta) -> [CAN5_FD_DKC_VehData_Sta]
  FDTBOXDTCDataErr/1(CAN5_FD_TBOX_DTCData_Err) -> [CAN5_FD_TBOX_DTCData_Err]
  FDTBOXDTCDataSta/1(CAN5_FD_TBOX_DTCData_Sta) -> [CAN5_FD_TBOX_DTCData_Sta]
  FDTBOXVehDataErr/1(CAN5_FD_TBOX_VehData_Err) -> [CAN5_FD_TBOX_VehData_Err]
  FDTBOXVehDataSta/1(CAN5_FD_TBOX_VehData_Sta) -> [CAN5_FD_TBOX_VehData_Sta]
  SWCmodeSta/1(CAN5_SWC_mode_Sta) -> [CAN5_SWC_mode_Sta]
  bus_selector/1 -> CCUAutoLampSts/1(CCUAutoLampSts)  "<VOUTP_CCUAutoLampSts_flg>"
  [BOUTP_outputs] -> bus_selector/1
  Ground/1 -> FDDKCVehDataErr/1(FDDKCVehDataErr)
  Ground1/1 -> FDDKCVehDataSta/1(FDDKCVehDataSta)
  Ground2/1 -> FDTBOXDTCDataErr/1(FDTBOXDTCDataErr)
  Ground3/1 -> FDTBOXDTCDataSta/1(FDTBOXDTCDataSta)
  Ground4/1 -> FDTBOXVehDataErr/1(FDTBOXVehDataErr)
  Ground5/1 -> FDTBOXVehDataSta/1(FDTBOXVehDataSta)
  bus_selector1/1 -> SWCmodeSta/1(SWCmodeSta)  "<VSCP_CAN5FDCONN1SWCmodeSta_flg>"
  [BSCP_outputs] -> bus_selector1/1

== system halout/HAL_OUT/CAN5/FD_THCM2_0x186 ==
  BSCP_outputs : Inport  OutDataTypeStr=Bus: BSCP_outputs
  BOUTP_outputs : Inport  Port=2  OutDataTypeStr=Bus: BOUTP_outputs
  ACSubMode : Subsystem
  APTCActFrRiPwr : Subsystem
  BatLoopActWtFlw : Subsystem
  CCUCbnPreACWkSts : Subsystem
  CCUCbnPreEstimdTi : Subsystem
  CCUCbnPreSts : Subsystem
  CCUHiVoltageReq : Subsystem
  CoolgFanActDuty : Subsystem
  DeiceModReq : Subsystem
  FDBlowerCmd : Subsystem
  FDCompCmd : Subsystem
  FDEWP1Cmd : Subsystem
  FDEWP2Cmd : Subsystem
  FDEWP3Cmd : Subsystem
  FDEXV1Cmd : Subsystem
  FDEXV2Cmd : Subsystem
  FDFWVCmd : Subsystem
  FDFrLeAPTCHeatPwrCmd : Subsystem
  FDFrRiAPTCHeatPwrCmd : Subsystem
  FDFrWPTCHeatPwrCmd : Subsystem
  FDRrAPTCHeatPwrCmd : Subsystem
  FDSOTXVCmd : Subsystem
  FDSOV1Cmd : Subsystem
  FDSOV2Cmd : Subsystem
  FDSOV3Cmd : Subsystem
  FDTWVCmd : Subsystem
  Ground{,1..6} (7 alike) : Ground
  bus_creator : BusCreator  Inputs=26  OutDataTypeStr=Bus: DT_CAN5_SG_FD_THCM2  NonVirtualBus=on
  bus_selector : BusSelector  OutputSignals=VOUTP_ACSubMode_enum
  bus_selector1 : BusSelector  OutputSignals=VOUTP_CoolgFanActDuty_pct
  bus_selector10 : BusSelector  OutputSignals=VOUTP_FDFrLeAPTCHeatPwrCmd_W
  bus_selector11 : BusSelector  OutputSignals=VOUTP_FDFrRiAPTCHeatPwrCmd_W
  bus_selector12 : BusSelector  OutputSignals=VOUTP_FDFrWPTCHeatPwrCmd_W
  bus_selector13 : BusSelector  OutputSignals=VOUTP_FDRrAPTCHeatPwrCmd_W
  bus_selector14 : BusSelector  OutputSignals=VOUTP_FDSOTXVCmd_flg
  bus_selector15 : BusSelector  OutputSignals=VOUTP_FDSOV1Cmd_flg
  bus_selector16 : BusSelector  OutputSignals=VOUTP_FDSOV2Cmd_flg
  bus_selector17 : BusSelector  OutputSignals=VOUTP_FDSOV3Cmd_flg
  bus_selector18 : BusSelector  OutputSignals=VOUTP_FDTWVCmd_pct
  bus_selector2 : BusSelector  OutputSignals=VOUTP_FDBlowerCmd_pct
  bus_selector3 : BusSelector  OutputSignals=VOUTP_FDCompCmd_rpm
  bus_selector4 : BusSelector  OutputSignals=VOUTP_FDEWP1Cmd_enum
  bus_selector5 : BusSelector  OutputSignals=VOUTP_FDEWP2Cmd_enum
  bus_selector6 : BusSelector  OutputSignals=VOUTP_FDEWP3Cmd_enum
  bus_selector7 : BusSelector  OutputSignals=VOUTP_FDEXV1Cmd_step
  bus_selector8 : BusSelector  OutputSignals=VOUTP_FDEXV2Cmd_step
  bus_selector9 : BusSelector  OutputSignals=VOUTP_FDFWVCmd_flg
  FD_THCM2 : Outport
  wires:
  BSCP_outputs/1 -> [BSCP_outputs]
  BOUTP_outputs/1 -> [BOUTP_outputs]
  [CAN5_ACSubMode] -> bus_creator/1  "CAN5_ACSubMode"
  [CAN5_APTC_ActFrRiPwr] -> bus_creator/2  "CAN5_APTC_ActFrRiPwr"
  [CAN5_BatLoopActWtFlw] -> bus_creator/3  "CAN5_BatLoopActWtFlw"
  [CAN5_CCU_CbnPreACWkSts] -> bus_creator/4  "CAN5_CCU_CbnPreACWkSts"
  [CAN5_CCU_CbnPreEstimdTi] -> bus_creator/5  "CAN5_CCU_CbnPreEstimdTi"
  [CAN5_CCU_CbnPreSts] -> bus_creator/6  "CAN5_CCU_CbnPreSts"
  [CAN5_CCU_HiVoltageReq] -> bus_creator/7  "CAN5_CCU_HiVoltageReq"
  [CAN5_CoolgFanActDuty] -> bus_creator/8  "CAN5_CoolgFanActDuty"
  [CAN5_DeiceModReq] -> bus_creator/9  "CAN5_DeiceModReq"
  [CAN5_FD_Blower_Cmd] -> bus_creator/10  "CAN5_FD_Blower_Cmd"
  [CAN5_FD_Comp_Cmd] -> bus_creator/11  "CAN5_FD_Comp_Cmd"
  [CAN5_FD_EWP1_Cmd] -> bus_creator/12  "CAN5_FD_EWP1_Cmd"
  [CAN5_FD_EWP2_Cmd] -> bus_creator/13  "CAN5_FD_EWP2_Cmd"
  [CAN5_FD_EWP3_Cmd] -> bus_creator/14  "CAN5_FD_EWP3_Cmd"
  [CAN5_FD_EXV1_Cmd] -> bus_creator/15  "CAN5_FD_EXV1_Cmd"
  [CAN5_FD_EXV2_Cmd] -> bus_creator/16  "CAN5_FD_EXV2_Cmd"
  [CAN5_FD_FWV_Cmd] -> bus_creator/17  "CAN5_FD_FWV_Cmd"
  [CAN5_FD_FrLeAPTCHeatPwr_Cmd] -> bus_creator/18  "CAN5_FD_FrLeAPTCHeatPwr_Cmd"
  [CAN5_FD_FrRiAPTCHeatPwr_Cmd] -> bus_creator/19  "CAN5_FD_FrRiAPTCHeatPwr_Cmd"
  [CAN5_FD_FrWPTCHeatPwr_Cmd] -> bus_creator/20  "CAN5_FD_FrWPTCHeatPwr_Cmd"
  [CAN5_FD_RrAPTCHeatPwr_Cmd] -> bus_creator/21  "CAN5_FD_RrAPTCHeatPwr_Cmd"
  [CAN5_FD_SOTXV_Cmd] -> bus_creator/22  "CAN5_FD_SOTXV_Cmd"
  [CAN5_FD_SOV1_Cmd] -> bus_creator/23  "CAN5_FD_SOV1_Cmd"
  [CAN5_FD_SOV2_Cmd] -> bus_creator/24  "CAN5_FD_SOV2_Cmd"
  [CAN5_FD_SOV3_Cmd] -> bus_creator/25  "CAN5_FD_SOV3_Cmd"
  [CAN5_FD_TWV_Cmd] -> bus_creator/26  "CAN5_FD_TWV_Cmd"
  bus_creator/1 -> FD_THCM2/1
  ACSubMode/1(CAN5_ACSubMode) -> [CAN5_ACSubMode]
  APTCActFrRiPwr/1(CAN5_APTC_ActFrRiPwr) -> [CAN5_APTC_ActFrRiPwr]
  BatLoopActWtFlw/1(CAN5_BatLoopActWtFlw) -> [CAN5_BatLoopActWtFlw]
  CCUCbnPreACWkSts/1(CAN5_CCU_CbnPreACWkSts) -> [CAN5_CCU_CbnPreACWkSts]
  CCUCbnPreEstimdTi/1(CAN5_CCU_CbnPreEstimdTi) -> [CAN5_CCU_CbnPreEstimdTi]
  CCUCbnPreSts/1(CAN5_CCU_CbnPreSts) -> [CAN5_CCU_CbnPreSts]
  CCUHiVoltageReq/1(CAN5_CCU_HiVoltageReq) -> [CAN5_CCU_HiVoltageReq]
  CoolgFanActDuty/1(CAN5_CoolgFanActDuty) -> [CAN5_CoolgFanActDuty]
  DeiceModReq/1(CAN5_DeiceModReq) -> [CAN5_DeiceModReq]
  FDBlowerCmd/1(CAN5_FD_Blower_Cmd) -> [CAN5_FD_Blower_Cmd]
  FDCompCmd/1(CAN5_FD_Comp_Cmd) -> [CAN5_FD_Comp_Cmd]
  FDEWP1Cmd/1(CAN5_FD_EWP1_Cmd) -> [CAN5_FD_EWP1_Cmd]
  FDEWP2Cmd/1(CAN5_FD_EWP2_Cmd) -> [CAN5_FD_EWP2_Cmd]
  FDEWP3Cmd/1(CAN5_FD_EWP3_Cmd) -> [CAN5_FD_EWP3_Cmd]
  FDEXV1Cmd/1(CAN5_FD_EXV1_Cmd) -> [CAN5_FD_EXV1_Cmd]
  FDEXV2Cmd/1(CAN5_FD_EXV2_Cmd) -> [CAN5_FD_EXV2_Cmd]
  FDFWVCmd/1(CAN5_FD_FWV_Cmd) -> [CAN5_FD_FWV_Cmd]
  FDFrLeAPTCHeatPwrCmd/1(CAN5_FD_FrLeAPTCHeatPwr_Cmd) -> [CAN5_FD_FrLeAPTCHeatPwr_Cmd]
  FDFrRiAPTCHeatPwrCmd/1(CAN5_FD_FrRiAPTCHeatPwr_Cmd) -> [CAN5_FD_FrRiAPTCHeatPwr_Cmd]
  FDFrWPTCHeatPwrCmd/1(CAN5_FD_FrWPTCHeatPwr_Cmd) -> [CAN5_FD_FrWPTCHeatPwr_Cmd]
  FDRrAPTCHeatPwrCmd/1(CAN5_FD_RrAPTCHeatPwr_Cmd) -> [CAN5_FD_RrAPTCHeatPwr_Cmd]
  FDSOTXVCmd/1(CAN5_FD_SOTXV_Cmd) -> [CAN5_FD_SOTXV_Cmd]
  FDSOV1Cmd/1(CAN5_FD_SOV1_Cmd) -> [CAN5_FD_SOV1_Cmd]
  FDSOV2Cmd/1(CAN5_FD_SOV2_Cmd) -> [CAN5_FD_SOV2_Cmd]
  FDSOV3Cmd/1(CAN5_FD_SOV3_Cmd) -> [CAN5_FD_SOV3_Cmd]
  FDTWVCmd/1(CAN5_FD_TWV_Cmd) -> [CAN5_FD_TWV_Cmd]
  bus_selector/1 -> ACSubMode/1(ACSubMode)  "<VOUTP_ACSubMode_enum>"
  [BOUTP_outputs] -> bus_selector/1
  Ground/1 -> APTCActFrRiPwr/1(APTCActFrRiPwr)
  Ground1/1 -> BatLoopActWtFlw/1(BatLoopActWtFlw)
  Ground2/1 -> CCUCbnPreACWkSts/1(CCUCbnPreACWkSts)
  Ground3/1 -> CCUCbnPreEstimdTi/1(CCUCbnPreEstimdTi)
  Ground4/1 -> CCUCbnPreSts/1(CCUCbnPreSts)
  Ground5/1 -> CCUHiVoltageReq/1(CCUHiVoltageReq)
  bus_selector1/1 -> CoolgFanActDuty/1(CoolgFanActDuty)  "<VOUTP_CoolgFanActDuty_pct>"
  [BOUTP_outputs] -> bus_selector1/1
  Ground6/1 -> DeiceModReq/1(DeiceModReq)
  bus_selector2/1 -> FDBlowerCmd/1(FDBlowerCmd)  "<VOUTP_FDBlowerCmd_pct>"
  [BOUTP_outputs] -> bus_selector2/1
  bus_selector3/1 -> FDCompCmd/1(FDCompCmd)  "<VOUTP_FDCompCmd_rpm>"
  [BOUTP_outputs] -> bus_selector3/1
  bus_selector4/1 -> FDEWP1Cmd/1(FDEWP1Cmd)  "<VOUTP_FDEWP1Cmd_enum>"
  [BOUTP_outputs] -> bus_selector4/1
  bus_selector5/1 -> FDEWP2Cmd/1(FDEWP2Cmd)  "<VOUTP_FDEWP2Cmd_enum>"
  [BOUTP_outputs] -> bus_selector5/1
  bus_selector6/1 -> FDEWP3Cmd/1(FDEWP3Cmd)  "<VOUTP_FDEWP3Cmd_enum>"
  [BOUTP_outputs] -> bus_selector6/1
  bus_selector7/1 -> FDEXV1Cmd/1(FDEXV1Cmd)  "<VOUTP_FDEXV1Cmd_step>"
  [BOUTP_outputs] -> bus_selector7/1
  bus_selector8/1 -> FDEXV2Cmd/1(FDEXV2Cmd)  "<VOUTP_FDEXV2Cmd_step>"
  [BOUTP_outputs] -> bus_selector8/1
  bus_selector9/1 -> FDFWVCmd/1(FDFWVCmd)  "<VOUTP_FDFWVCmd_flg>"
  [BOUTP_outputs] -> bus_selector9/1
  bus_selector10/1 -> FDFrLeAPTCHeatPwrCmd/1(FDFrLeAPTCHeatPwrCmd)  "<VOUTP_FDFrLeAPTCHeatPwrCmd_W>"
  [BOUTP_outputs] -> bus_selector10/1
  bus_selector11/1 -> FDFrRiAPTCHeatPwrCmd/1(FDFrRiAPTCHeatPwrCmd)  "<VOUTP_FDFrRiAPTCHeatPwrCmd_W>"
  [BOUTP_outputs] -> bus_selector11/1
  bus_selector12/1 -> FDFrWPTCHeatPwrCmd/1(FDFrWPTCHeatPwrCmd)  "<VOUTP_FDFrWPTCHeatPwrCmd_W>"
  [BOUTP_outputs] -> bus_selector12/1
  bus_selector13/1 -> FDRrAPTCHeatPwrCmd/1(FDRrAPTCHeatPwrCmd)  "<VOUTP_FDRrAPTCHeatPwrCmd_W>"
  [BOUTP_outputs] -> bus_selector13/1
  bus_selector14/1 -> FDSOTXVCmd/1(FDSOTXVCmd)  "<VOUTP_FDSOTXVCmd_flg>"
  [BOUTP_outputs] -> bus_selector14/1
  bus_selector15/1 -> FDSOV1Cmd/1(FDSOV1Cmd)  "<VOUTP_FDSOV1Cmd_flg>"
  [BOUTP_outputs] -> bus_selector15/1
  bus_selector16/1 -> FDSOV2Cmd/1(FDSOV2Cmd)  "<VOUTP_FDSOV2Cmd_flg>"
  [BOUTP_outputs] -> bus_selector16/1
  bus_selector17/1 -> FDSOV3Cmd/1(FDSOV3Cmd)  "<VOUTP_FDSOV3Cmd_flg>"
  [BOUTP_outputs] -> bus_selector17/1
  bus_selector18/1 -> FDTWVCmd/1(FDTWVCmd)  "<VOUTP_FDTWVCmd_pct>"
  [BOUTP_outputs] -> bus_selector18/1
